simulink model "DiagramaDeSimulacaoItem5"  (R2018a)
settings: Solver=VariableStepAuto  StartTime=0.0  StopTime=10  RelTol=1e-3
values from neighbouring files (symbols this model uses):
  CaEq = 0.7192    [scriptItem5.m]
  CafEq = 5.1    [scriptItem5.m]
  CbEq = 2.345    [scriptItem5.m]
  k1 = 6.01    [Q5.m]    (also in scriptItem5.m)
  k2 = 0.8433    [Q5.m]    (also in scriptItem5.m)
  k3 = 0.1123    [Q5.m]    (also in scriptItem5.m)
  uEq = 1    [scriptItem5.m]
settings Model: Creator=Usuario  LastModifiedBy=crist
settings DataIOCC: ReturnWorkspaceOutputs=on
settings SFSimCC: SimUseLocalCustomCode=on
settings RTWCC: RTWUseLocalCustomCode=on

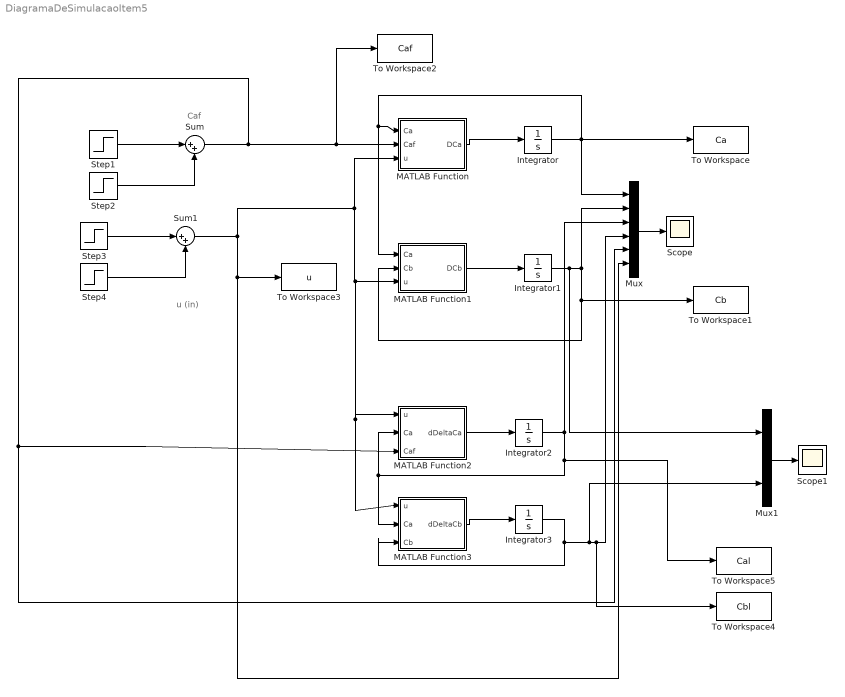
== system DiagramaDeSimulacaoItem5 ==
  note: u (in)
  note: Caf
  Integrator : Integrator  InitialCondition=0.7192
  Integrator1 : Integrator  InitialCondition=2.345
  Integrator2 : Integrator  InitialCondition=0.7192
  Integrator3 : Integrator  InitialCondition=2.345
  MATLAB Function : MATLAB Function  TreatAsAtomicUnit=on
  MATLAB Function1 : MATLAB Function  TreatAsAtomicUnit=on
  MATLAB Function2 : MATLAB Function  TreatAsAtomicUnit=on
  MATLAB Function3 : MATLAB Function  TreatAsAtomicUnit=on
  Mux : Mux  Inputs=6
  Mux1 : Mux  Inputs=2
  Scope : Scope
  Scope1 : Scope
  Step1 : Step  Time=2.5  Before=5.1  After=5.6  SampleTime=0
  Step2 : Step  Time=7.5  After=0.5  SampleTime=0
  Step3 : Step  Time=2.5  Before=1  After=1.05  SampleTime=0
  Step4 : Step  Time=7.5  After=0.2  SampleTime=0
  Sum : Sum  Inputs=|++
  Sum1 : Sum  Inputs=|++
  To Workspace : ToWorkspace  VariableName=Ca  SaveFormat=Timeseries  SampleTime=-1
  To Workspace1 : ToWorkspace  VariableName=Cb  SaveFormat=Timeseries  SampleTime=-1
  To Workspace2 : ToWorkspace  VariableName=Caf  SaveFormat=Timeseries  SampleTime=-1
  To Workspace3 : ToWorkspace  VariableName=u  SaveFormat=Timeseries  SampleTime=-1
  To Workspace4 : ToWorkspace  VariableName=Cbl  SaveFormat=Timeseries  SampleTime=-1
  To Workspace5 : ToWorkspace  VariableName=Cal  SaveFormat=Timeseries  SampleTime=-1
  wires:
  MATLAB Function/1(DCa) -> Integrator/1
  MATLAB Function1/1(DCb) -> Integrator1/1
  Integrator/1 -> To Workspace/1, Mux/1, MATLAB Function1/1(Ca), MATLAB Function/1(Ca)
  Integrator1/1 -> Mux1/1, To Workspace1/1, MATLAB Function1/2(Cb), Mux/2
  Mux/1 -> Scope/1
  Sum1/1 -> MATLAB Function/3(u), MATLAB Function3/1(u), MATLAB Function2/1(u), MATLAB Function1/3(u), To Workspace3/1, Mux/6
  Sum/1 -> To Workspace2/1, MATLAB Function/2(Caf), MATLAB Function2/3(Caf), Mux/5
  MATLAB Function2/1(dDeltaCa) -> Integrator2/1
  MATLAB Function3/1(dDeltaCb) -> Integrator3/1
  Integrator2/1 -> To Workspace5/1, MATLAB Function3/2(Ca), MATLAB Function2/2(Ca), Mux/3
  Integrator3/1 -> Mux1/2, To Workspace4/1, Mux/4, MATLAB Function3/3(Cb)
  Step1/1 -> Sum/1
  Step2/1 -> Sum/2
  Step4/1 -> Sum1/2
  Step3/1 -> Sum1/1
  Mux1/1 -> Scope1/1

== matlab function DiagramaDeSimulacaoItem5/MATLAB Function1 ==
  data: DCb output; Ca input; Cb input; u input; k2 parameter; k1 parameter
function DCb = fcn(Ca,Cb,u, k2, k1)

DCb = k1*Ca - k2*Cb - Cb*u;

== matlab function DiagramaDeSimulacaoItem5/MATLAB Function ==
  data: DCa output; Ca input; Caf input; k1 parameter; k3 parameter; u input
function DCa = fcn(Ca,Caf,k1, k3, u)

DCa = -k1*Ca - k3*Ca^2 + (Caf -Ca)*u;

== matlab function DiagramaDeSimulacaoItem5/MATLAB Function2 ==
  data: u input; dDeltaCa output; Ca input; Caf input; CaEq parameter; k1 parameter; k3 parameter; uEq parameter; CafEq parameter
function dDeltaCa = fcn(u,Ca,Caf, CaEq, k1, k3, uEq, CafEq)

dDeltaCa = (Ca-CaEq)*(-k1-2*k3*CaEq - uEq) + (u-uEq)*(CafEq-CaEq) + (Caf-CafEq)*uEq;

== matlab function DiagramaDeSimulacaoItem5/MATLAB Function3 ==
  data: u input; dDeltaCb output; Ca input; CaEq parameter; k1 parameter; k2 parameter; uEq parameter; Cb input; CbEq parameter
function dDeltaCb = fcn(u,Ca, CaEq, k1, k2, uEq, Cb, CbEq)

dDeltaCb = (Ca-CaEq)*(k1) + (Cb-CbEq)*(-uEq-k2) + (u-uEq)*(-CbEq);
